simulink model "PMSM_FOC_sensorless"  (R2026a)
settings: Solver=FixedStepDiscrete  StopTime=10  FixedStep=Ts  EnableMultiTasking=on
InitFcn:
  | ParameterInit
undefined symbols (not defined in the file): drive, FAKF, motor, Ts
libraries: simulink x10, mcbhdlcontrolslib x10, matrix_library x8, mcbcontrolslib x6, mcbpositiondecoderlib x3, mcbsensorlessestimatorlib x2, mcbeeMathTransformLib x2, slpidlib x2, sl_discontinuities x1, mcbplantlib x1, autolibpmsminterior x1, realtime_pacer_lib x1
(part 3 of 3)

== system PMSM_FOC_sensorless/FOC/Observer/对比观测器/EKF/angle limit1 ==
  θ : Inport
  Constant2 : Constant  Value=-pi  OutDataTypeStr=single
  Constant4 : Constant  Value=pi  OutDataTypeStr=single
  Demux : Demux
  Gain6 : Gain  Gain=-2*pi  OutDataTypeStr=single
  Gain7 : Gain  Gain=2*pi  OutDataTypeStr=single
  Mux : Mux
  Relational Operator2 : RelationalOperator  Operator=<  RndMeth=Simplest  InputSameDT=off
  Relational Operator3 : RelationalOperator  Operator=<=  RndMeth=Simplest  InputSameDT=off
  Sum3 : Sum  Inputs=+++
  "[-pi,pi)" : Outport
  wires:
  Demux/1 -> Mux/1
  Mux/1 -> "[-pi,pi)"/1
  θ/1 -> Demux/1
  Sum3/1 -> Mux/4
  Gain6/1 -> Sum3/1
  Relational Operator2/1 -> Gain7/1
  Gain7/1 -> Sum3/3
  Relational Operator3/1 -> Gain6/1
  Constant4/1 -> Relational Operator3/1
  Demux/4 -> Relational Operator2/1, Sum3/2, Relational Operator3/2
  Constant2/1 -> Relational Operator2/2
  Demux/3 -> Mux/3
  Demux/2 -> Mux/2

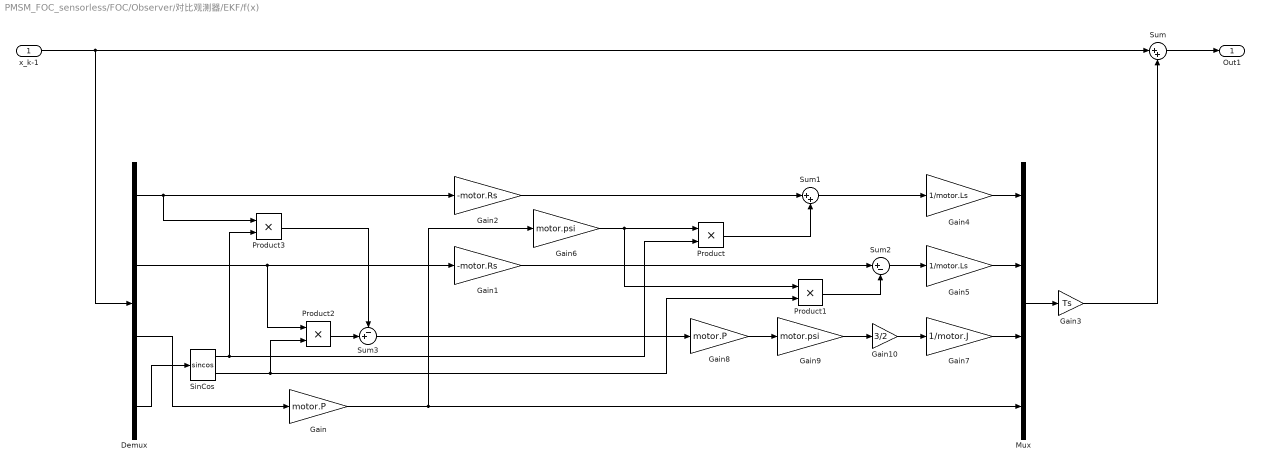
== system PMSM_FOC_sensorless/FOC/Observer/对比观测器/EKF/f(x) ==
  x_k-1 : Inport
  Demux : Demux
  Gain : Gain  Gain=motor.P
  Gain1 : Gain  Gain=-motor.Rs
  Gain10 : Gain  Gain=3/2
  Gain2 : Gain  Gain=-motor.Rs
  Gain3 : Gain  Gain=Ts
  Gain4 : Gain  Gain=1/motor.Ls
  Gain5 : Gain  Gain=1/motor.Ls
  Gain6 : Gain  Gain=motor.psi
  Gain7 : Gain  Gain=1/motor.J
  Gain8 : Gain  Gain=motor.P
  Gain9 : Gain  Gain=motor.psi
  Mux : Mux
  Product{,1..3} (4 alike) : Product
  SinCos : Trigonometry  Operator=sincos
  Sum : Sum  Inputs=|++
  Sum1 : Sum  Inputs=|++
  Sum2 : Sum  Inputs=|+-
  Sum3 : Sum  Inputs=-+|
  Out1 : Outport
  wires:
  x_k-1/1 -> Demux/1, Sum/1
  Mux/1 -> Gain3/1
  Demux/1 -> Gain2/1, Product3/1
  Gain2/1 -> Sum1/1
  Demux/2 -> Gain1/1, Product2/1
  Gain1/1 -> Sum2/1
  Sum1/1 -> Gain4/1
  Sum2/1 -> Gain5/1
  Gain3/1 -> Sum/2
  Gain4/1 -> Mux/1
  Gain5/1 -> Mux/2
  Demux/4 -> SinCos/1
  Gain7/1 -> Mux/3
  Demux/3 -> Gain/1
  Sum/1 -> Out1/1
  Gain/1 -> Gain6/1, Mux/4
  Product/1 -> Sum1/2
  Gain6/1 -> Product1/1, Product/1
  SinCos/1 -> Product/2, Product3/2
  Product1/1 -> Sum2/2
  SinCos/2 -> Product1/2, Product2/2
  Gain8/1 -> Gain9/1
  Gain10/1 -> Gain7/1
  Gain9/1 -> Gain10/1
  Product2/1 -> Sum3/2
  Product3/1 -> Sum3/1
  Sum3/1 -> Gain8/1

== system PMSM_FOC_sensorless/FOC/Observer/对比观测器/FKF/AKF ==
  u_k : Inport
  z_k : Inport  Port=2
  Constant1 : Constant  Value=[0.1421,-0.077657;0.0001717,0.002415]  VectorParams1D=off  OutDataTypeStr=single
  Constant4 : Constant  Value=[0.3508,7.253;0.000117,0.0586]  VectorParams1D=off  OutDataTypeStr=single
  状态观测 : Subsystem
  x_k : Outport
  wires:
  u_k/1 -> 状态观测/1(u)
  z_k/1 -> 状态观测/2(z)
  状态观测/1(x^) -> x_k/1  "x^"
  Constant4/1 -> 状态观测/3(K)  "K"

== system PMSM_FOC_sensorless/FOC/Observer/对比观测器/FKF/位置提取 ==
  Eαβ : Inport
  θ_sincos : Inport  Port=2
  Constant : Constant  Value=motor.psi  OutDataTypeStr=single
  Demux : Demux  Outputs=2
  Divide3 : Product  Inputs=/*
  Gain : Gain  Gain=[-1 1]  Multiplication=Matrix(K*u)
  Gain1 : Gain  Gain=motor.P
  Gain2 : Gain  Gain=-1
  Mux : Mux  Inputs=2
  Product : Product
  Product1 : Product
  Sign : Signum
  Unit Delay : UnitDelay  SampleTime=-1
  幅角 : mcbcontrolslib/atan2  ApproximationMethod=None  NumberOfIterations=11  NumberOfDataPoints=16  InterpMethod=Flat  outputUnit=Radians  TableDataTypeStr=Inherit: Inherit via input
  ωθ : Outport
  wires:
  Constant/1 -> Gain1/1
  Gain1/1 -> Divide3/1
  幅角/1 -> Mux/2
  θ_sincos/1 -> Unit Delay/1
  Unit Delay/1 -> Product/1
  Product/1 -> Gain/1
  Gain/1 -> Divide3/2, Sign/1
  Divide3/1 -> Mux/1
  Mux/1 -> ωθ/1
  Demux/2 -> 幅角/2
  Demux/1 -> Gain2/1
  Gain2/1 -> 幅角/1
  Eαβ/1 -> Product/2, Product1/2
  Sign/1 -> Product1/1
  Product1/1 -> Demux/1

== system PMSM_FOC_sensorless/FOC/Observer/对比观测器/FKF/角度转换 ==
  θ : Inport
  Mux1 : Mux  Inputs=2
  SinCos : Trigonometry  Operator=sincos
  sincos : Outport
  wires:
  SinCos/1 -> Mux1/1
  θ/1 -> SinCos/1
  SinCos/2 -> Mux1/2
  Mux1/1 -> sincos/1

== system PMSM_FOC_sensorless/FOC/Observer/对比观测器/FKF/计算转子反电动势 ==
  Iαβ : Inport
  Uαβ : Inport  Port=2
  Sum5 : Sum  Inputs=+--
  滞后补偿 : DiscreteFilter  Numerator=[0 0 1 1]  Denominator=[2 0 0 0]
  电感分压 : simulink/Discrete/Discrete Derivative  gainval=motor.Ls  ICPrevScaledInput=0.0  OutMin=[]  OutMax=[]  OutDataType=fixdt(1, 16)  OutScaling=2^-10  DoSatur=off
  电阻分压 : Gain  Gain=motor.Rs
  Eαβ : Outport
  wires:
  电感分压/1 -> Sum5/3
  电阻分压/1 -> Sum5/2
  Uαβ/1 -> 滞后补偿/1
  Iαβ/1 -> 电感分压/1, 电阻分压/1
  滞后补偿/1 -> Sum5/1
  Sum5/1 -> Eαβ/1

== system PMSM_FOC_sensorless/FOC/Observer/对比观测器/FKF/转矩计算 ==
  θ_sincos : Inport
  I_αβ : Inport  Port=2
  Constant : Constant  Value=motor.psi  OutDataTypeStr=single
  Divide1 : Product  Inputs=**
  Gain : Gain  Gain=[-1 1]  Multiplication=Matrix(K*u)
  Gain1 : Gain  Gain=motor.P
  Gain2 : Gain  Gain=1.5
  Product3 : Product
  Unit Delay : UnitDelay  SampleTime=-1
  T : Outport
  wires:
  Product3/1 -> Gain/1
  Constant/1 -> Gain1/1
  Divide1/1 -> Gain2/1
  Gain/1 -> Divide1/1
  Unit Delay/1 -> Product3/1
  I_αβ/1 -> Product3/2
  θ_sincos/1 -> Unit Delay/1
  Gain1/1 -> Divide1/2
  Gain2/1 -> T/1

== system PMSM_FOC_sensorless/FOC/Observer/对比观测器/FKF/AKF/状态观测 ==
  note: 预测状态
  note: 计算残差
  note: 更新最优状态
  u : Inport
  z : Inport  Port=2
  K : Inport  Port=3
  Divide4 : Product  Inputs=**  Multiplication=Matrix(*)
  Gain : Gain  Gain=[1-motor.damp*Ts/motor.J,0;motor.P*Ts,1]  Multiplication=Matrix(K*u)
  Gain1 : Gain  Gain=[Ts/motor.J;0]  Multiplication=Matrix(K*u)
  Gain2 : Gain  Gain=[motor.J/Ts 0]  Multiplication=Matrix(K*u)
  Sum : Sum  Inputs=+|+
  Sum1 : Sum  Inputs=-+|
  Sum2 : Sum  Inputs=-+|
  Sum3 : Sum  Inputs=|++
  Unit Delay2 : UnitDelay  SampleTime=-1
  angle limit1 : Subsystem
  angle limit3 : Subsystem
  摩擦转矩补偿 : Saturate  UpperLimit=motor.fric  LowerLimit=-motor.fric
  x^ : Outport
  wires:
  Sum/1 -> Sum2/1, Sum3/1
  angle limit1/1(P_k1) -> Divide4/2
  Sum3/1 -> angle limit3/1(In)
  Gain1/1 -> Sum/1
  Gain/1 -> Sum/2
  Unit Delay2/1 -> Gain2/1, Gain/1
  Divide4/1 -> Sum3/2
  Sum1/1 -> Gain1/1
  Gain2/1 -> 摩擦转矩补偿/1
  angle limit3/1(x) -> x^/1, Unit Delay2/1
  Sum2/1 -> angle limit1/1(In)
  u/1 -> Sum1/2
  z/1 -> Sum2/2
  K/1 -> Divide4/1
  摩擦转矩补偿/1 -> Sum1/1  "dir3"

== system PMSM_FOC_sensorless/FOC/Observer/对比观测器/FKF/AKF/状态观测/angle limit1 ==
  In : Inport
  Constant2 : Constant  Value=-pi  OutDataTypeStr=single
  Constant4 : Constant  Value=pi  OutDataTypeStr=single
  Demux : Demux  Outputs=2
  Gain6 : Gain  Gain=-2*pi  OutDataTypeStr=single
  Gain7 : Gain  Gain=2*pi  OutDataTypeStr=single
  Mux : Mux  Inputs=2
  Relational Operator2 : RelationalOperator  Operator=<  RndMeth=Simplest  InputSameDT=off
  Relational Operator3 : RelationalOperator  Operator=<  RndMeth=Simplest  InputSameDT=off
  Sum3 : Sum  Inputs=+++
  P_k1 : Outport
  wires:
  Demux/1 -> Mux/1
  Mux/1 -> P_k1/1
  In/1 -> Demux/1
  Sum3/1 -> Mux/2
  Gain6/1 -> Sum3/1
  Relational Operator2/1 -> Gain7/1
  Gain7/1 -> Sum3/3
  Relational Operator3/1 -> Gain6/1
  Constant4/1 -> Relational Operator3/1
  Demux/2 -> Relational Operator2/1, Sum3/2, Relational Operator3/2
  Constant2/1 -> Relational Operator2/2

== system PMSM_FOC_sensorless/FOC/Observer/对比观测器/FKF/AKF/状态观测/angle limit3 ==
  In : Inport
  Constant2 : Constant  Value=-pi  OutDataTypeStr=single
  Constant4 : Constant  Value=pi  OutDataTypeStr=single
  Demux : Demux  Outputs=2
  Gain6 : Gain  Gain=-2*pi  OutDataTypeStr=single
  Gain7 : Gain  Gain=2*pi  OutDataTypeStr=single
  Mux : Mux  Inputs=2
  Relational Operator2 : RelationalOperator  Operator=<  RndMeth=Simplest  InputSameDT=off
  Relational Operator3 : RelationalOperator  Operator=<  RndMeth=Simplest  InputSameDT=off
  Sum3 : Sum  Inputs=+++
  x : Outport
  wires:
  Constant2/1 -> Relational Operator2/2
  Demux/2 -> Relational Operator3/2, Sum3/2, Relational Operator2/1
  Constant4/1 -> Relational Operator3/1
  Relational Operator3/1 -> Gain6/1
  Gain7/1 -> Sum3/3
  Relational Operator2/1 -> Gain7/1
  Gain6/1 -> Sum3/1
  Sum3/1 -> Mux/2
  In/1 -> Demux/1
  Mux/1 -> x/1
  Demux/1 -> Mux/1

== matlab function PMSM_FOC_sensorless/控制面板/MATLAB Function ==
  data: t input; y output
function y = fcn(t)
    
    y_m = 1.2;
    if(t<1)
        y = 0;
    elseif(t<2)
        y = t-1;
    elseif(t<4)
        y = 3-t;
    elseif(t<5)
        y = t-5;
    else
        y=0;
    end
    y = y*y_m;
end

== matlab function PMSM_FOC_sensorless/数据可视化/卡尔曼过程可视化/协方差动态显示1 ==
  data: x_1 input; P_1 input; z input; R input; x input; P input; range input; en input
function fcn(x_1,P_1,z,R,x,P,range,en)

    % x_1(1,:) = abs(x_1(1,:));
    % x(1,:) = abs(x(1,:));
    % z(1,:) = abs(z(1,:));
    P_1 = point2cir(x_1(:,1),sqrtm(P_1));
    R = point2cir(z(:,1),sqrtm(R));
    P = point2cir(x(:,1),sqrtm(P));
    
    if(en == 1)
        x_1 = polar2xy(x_1);
        x = polar2xy(x);
        z = polar2xy(z);
        P_1 = polar2xy(P_1);
        P = polar2xy(P);
        R = polar2xy(R);

        hold off;
        plot(z(1,:), z(2,:),'c.-');
        hold on;
        plot(R(1,:),R(2,:),'c-','LineWidth', 2);

        plot(x_1(1,:),x_1(2,:),'gx');
        plot(P_1(1,:),P_1(2,:),'g-','LineWidth', 2);

        plot(x(1,:),x(2,:),'r.-');
        plot(P(1,:),P(2,:),'r-','LineWidth', 2);
        axis([-range, range,-range, range]);
        % 显示网格
        grid on;
        box off;
    elseif(en == 2)
        hold off;
        polarplot(z(2,:), z(1,:),'c-');
        hold on;
        polarplot(R(2,:),R(1,:),'c-','LineWidth', 2);

        polarplot(x_1(2,:), x_1(1,:),'gx');
        polarplot(P_1(2,:),P_1(1,:),'g-','LineWidth', 2);

        polarplot(x(2,:), x(1,:),'r-');
        polarplot(P(2,:),P(1,:),'r-','LineWidth', 2);
        axis([0,360,0, range]);
    elseif(en == 3)
        subplot(1, 2, 1);
        hold off;
        polarplot(z(2,:), z(1,:),'c-');
        hold on;
        polarplot(R(2,:),R(1,:),'c-','LineWidth', 2);

        polarplot(x_1(2,:), x_1(1,:),'gx');
        polarplot(P_1(2,:),P_1(1,:),'g-','LineWidth', 2);

        polarplot(x(2,:), x(1,:),'r-');
        polarplot(P(2,:),P(1,:),'r-','LineWidth', 2);
        axis([0,360,0, range]);
        title("\omega_m-\theta_e");

        subplot(1, 2, 2);
        x_1 = polar2xy(x_1);
        x = polar2xy(x);
        z = polar2xy(z);
        P_1 = polar2xy(P_1);
        P = polar2xy(P);
        R = polar2xy(R);

        hold off;
        plot(z(1,1:2), z(2,1:2),'c.-');
        hold on;
        plot(R(1,:),R(2,:),'c-','LineWidth', 2);

        plot(x_1(1,:),x_1(2,:),'gx');
        plot(P_1(1,:),P_1(2,:),'g-','LineWidth', 2);

        plot(x(1,1:2),x(2,1:2),'r.-');
        plot(P(1,:),P(2,:),'r-','LineWidth', 2);
        xlabel('\omega_{m,\alpha}(radps)','Interpreter', 'tex');
        ylabel('\omega_{m,\beta}(radps)','Interpreter', 'tex');
        axis([x(1,2)-10, x(1,2)+10,x(2,2)-10, x(2,2)+10]);
        title("Covariance matrix");
        legend({'','R_k', ...
                '','P_{k|k-1}', ...
                '','P_k'});
        % 显示网格
        grid on;
        box off;
    end
end

%% 均值位p,方差为C的随机变量分布范围
function y = point2cir(p,P)

    if(P == 0)
        y = p;
    else
        t = linspace(-pi,pi,64);
        cir = [cos(t);sin(t)];
        y = p + 2*(P)*cir;
    end
end

function y = polar2xy(u)
    y = [u(1,:).*cos(u(2,:));
         u(1,:).*sin(u(2,:))];
end

== matlab function PMSM_FOC_sensorless/数据可视化/卡尔曼过程可视化/Subsystem2/MATLAB Function ==
  data: u input; y output; y_1 input
function y = fcn(u, y_1)
    y = [u,y_1(:,1:end-1)];
end

== matlab function PMSM_FOC_sensorless/数据可视化/卡尔曼过程可视化/Subsystem1/MATLAB Function ==
  data: u input; y output; y_1 input
function y = fcn(u, y_1)
    y = [u,y_1(:,1:end-1)];
end
